simulink model "Solar_power_generation_for_home"  (R2020a)
settings: Solver=VariableStepAuto  StartTime=0.0  StopTime=10.0  RelTol=1e-3
libraries: powerlib x13, powerlib_meascontrol x1, re_lib x1
settings Model: Creator=Reaga  LastModifiedBy=Reaga
settings DebuggingCC: UnconnectedInputMsg=none  UnconnectedOutputMsg=none  UnconnectedLineMsg=none
settings ModelReferenceCC: EnableRefExpFcnMdlSchedulingChecks=off
settings RTWCC: Description=Generic Real-Time Target
settings ConfigComp: CovBoundaryAbsTol=1.0e-5

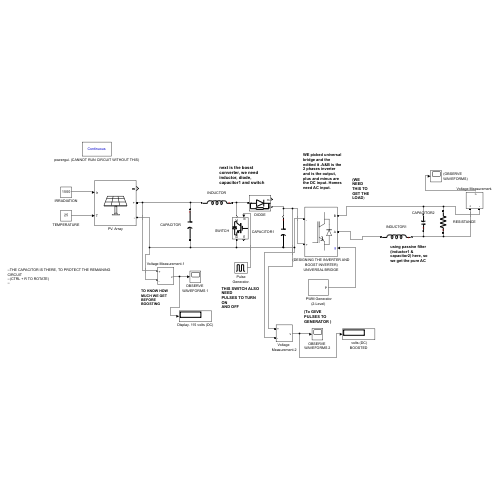
[thumbnail: Simulink's stored preview of the top-level diagram]
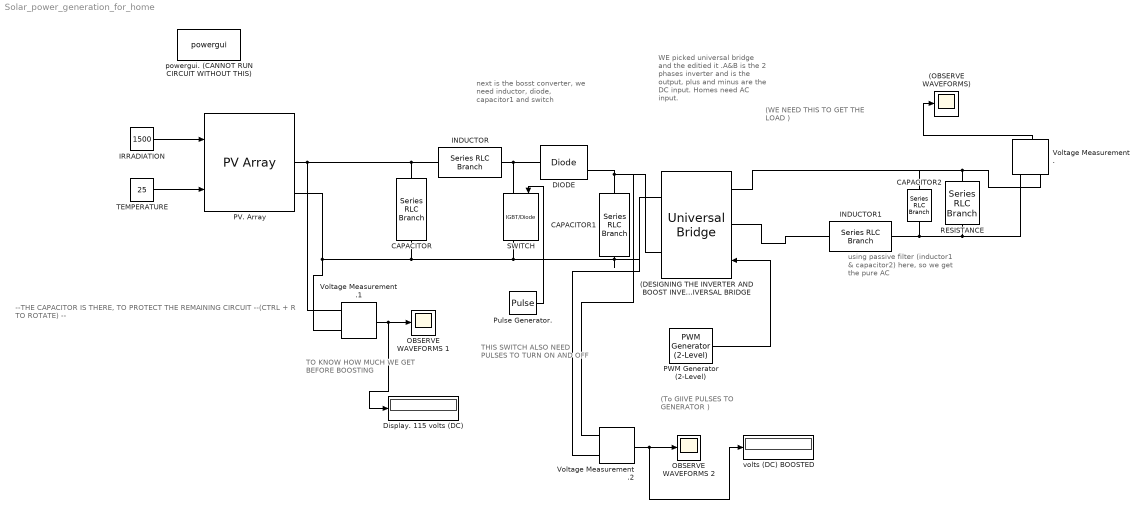
== system Solar_power_generation_for_home ==
  note: using passive filter (inductor1 & capacitor2) here, so we get the pure AC
  note: TO KNOW HOW MUCH WE GET
      | BEFORE BOOSTING
  note: THIS SWITCH ALSO NEED
      | PULSES TO TURN ON
      | AND OFF
  note: (To GIIVE PULSES TO GENERATOR )
  note: (WE NEED THIS TO
      | GET THE LOAD )
  note: WE picked universal bridge and the editied it .A&B is the 2 phases inverter and is the output, plus and minus are the DC input. Homes need AC input.
  note: next is the bosst converter, we need inductor, diode, capacitor1 and switch
  note: --THE CAPACITOR IS THERE, TO PROTECT THE REMAINING CIRCUIT
      | --(CTRL + R TO ROTATE)
      | --
  " SWITCH " : powerlib/Power Electronics/IGBT//Diode  Ron=1e-3  Rs=1e5  Cs=inf  Measurements=on
  " PWM Generator (2-Level)" : powerlib_meascontrol/Pulse & Signal Generators/PWM Generator (2-Level)  ModulatorType=Single-phase full-bridge (4 pulses)  ModulatorMode=Unsynchronized  Fc=27*60  Pc=90  nF=27  MinMax="[ -1  1 ]"  SamplingTechnique=Natural  ModulatingSignals=on  m=0.8  Freq=60  Phase=0  Ts=0  ShowCarrierOutport=off
  " volts (DC) BOOSTED" : Display
  (DESIGNING THE INVERTER AND BOOST INVERTER) UNIVERSAL BRIDGE : powerlib/Power Electronics/Universal Bridge  Arms=2  SnubberResistance=1e5  SnubberCapacitance=inf  Device=IGBT / Diodes  Ron=1e-3  Lon=0  ForwardVoltages="[  0  0  ]"  ForwardVoltage=0  GTOparameters=[ 10e-6 , 20e-6 ]  IGBTparameters=[ 1e-6 , 2e-6 ]  Measurements=None  Measurements_2=None  converterType=Rectifier
  (OBSERVE WAVEFORMS) : Scope
  CAPACITOR : powerlib/Elements/Series RLC Branch  LConnTagsString=__new0  RConnTagsString=__new0  BranchType=C  Resistance=1  Inductance=1e-3  SetiL0=off  InitialCurrent=0  Capacitance=0.006  Setx0=off  InitialVoltage=0  Measurements=None
  CAPACITOR1 : powerlib/Elements/Series RLC Branch  LConnTagsString=__new0  RConnTagsString=__new0  BranchType=C  Resistance=1  Inductance=1e-3  SetiL0=off  InitialCurrent=0  Capacitance=0.006  Setx0=off  InitialVoltage=0  Measurements=None
  CAPACITOR2 : powerlib/Elements/Series RLC Branch  LConnTagsString=__new0  RConnTagsString=__new0  BranchType=C  Resistance=1  Inductance=1e-3  SetiL0=off  InitialCurrent=0  Capacitance=0.006  Setx0=off  InitialVoltage=0  Measurements=None
  DIODE : powerlib/Power Electronics/Diode  Ron=0.001  Lon=0  Vf=0.8  IC=0  UseSnubber=0  Rs=500  Cs=250e-9  Measurements=on
  Display. 115 volts (DC) : Display
  INDUCTOR : powerlib/Elements/Series RLC Branch  LConnTagsString=__new0  RConnTagsString=__new0  BranchType=L  Resistance=1  Inductance=0.02  SetiL0=off  InitialCurrent=0  Capacitance=0.006  Setx0=off  InitialVoltage=0  Measurements=None
  INDUCTOR1 : powerlib/Elements/Series RLC Branch  LConnTagsString=__new0  RConnTagsString=__new0  BranchType=L  Resistance=1  Inductance=0.02  SetiL0=off  InitialCurrent=0  Capacitance=0.006  Setx0=off  InitialVoltage=0  Measurements=None
  IRRADIATION : Constant  Value=1500
  OBSERVE WAVEFORMS 1 : Scope
  OBSERVE WAVEFORMS 2 : Scope
  PV. Array : re_lib/Solar/PV Array  Npar=20  Nser=5  PlotType=array @ 1000 W/m2 & specified temperatures  S_vec="[ 1000  500  100 ]"  Temp_C_vec="[ 45 25  ]"  ModuleName=User-defined  PlotWhenSelected=off  Pm=213.15  Ncell=60  Voc=36.3  Isc=7.84  Vm=29  Im=7.35  beta_Voc_pc=-0.36099  alpha_Isc_pc=0.102  beta_Voc=-0.13104  alpha_Isc=0.0079968  IL=7.8654  I0=2.9273e-10  nI=0.98119  Rsh=313.0553  Rs=0.39381  RobustModel=off  RobustCellTemperature=313.3991  BAL=on  Tc=1e-6  Tfilter=5e-5
  Pulse Generator. : DiscretePulseGenerator  PulseType=Time based  Period=1/1500  PulseWidth=50
  RESISTANCE : powerlib/Elements/Series RLC Branch  LConnTagsString=__new0  RConnTagsString=__new0  BranchType=R  Resistance=1  Inductance=1e-3  SetiL0=off  InitialCurrent=0  Capacitance=0.006  Setx0=off  InitialVoltage=0  Measurements=None
  TEMPERATURE : Constant  Value=25
  Voltage Measurement.2 : powerlib/Measurements/Voltage Measurement  PhasorSimulation=off  OutputType=Complex  PSBequivalent=0
  Voltage Measurement. : powerlib/Measurements/Voltage Measurement  PhasorSimulation=off  OutputType=Complex  PSBequivalent=0
  Voltage Measurement.1 : powerlib/Measurements/Voltage Measurement  PhasorSimulation=off  OutputType=Complex  PSBequivalent=0
  powergui. (CANNOT RUN CIRCUIT WITHOUT THIS) : powerlib/powergui  Priority=1  SimulationMode=Continuous  SampleTime=50e-6  frequency=60  Iterations=50  frequencyindice=0  Pbase=100e6  ErrMax=1e-4  UnitsV=kV  UnitsW=MW  buscounter=0  FunctionMessages=off  echomessages=off  EnableUseOfTLC=off  CurrentSourceSwitches=off  DisableSnubberDevices=off  DisableRonSwitches=off  DisableVfSwitches=off  DisplayEquations=off  AutomaticDiscreteSolvers=off  SolverType=Tustin/Backward Euler (TBE)  Interpol=off  ExternalGateDelay=off  methode=off  Ts=100  x0status=blocks  SPID=on  SwTol=0  HookPort=off  NonlinearTolerance=1e-4  nMaxIteration=100  ContinueOnMaxIteration=off  RestoreLinks=warning  ResistiveCurrentMeasurement=off  Frange=[0:2:500]  Ylog=off  Xlog=on  ShowGrid=off  save=off  variable=ZData  structure=0  ZoomFFT=off  StartTime=0.0  cycles=1  DisplayStyle=1  fundamental=60  FreqAxis=off  MaxFrequency=1000  frequencyindicesteady=1  RmsSteady=1  display=off
  wires:
  TEMPERATURE/1 -> PV. Array/2
  IRRADIATION/1 -> PV. Array/1
  " PWM Generator (2-Level)"/1 -> (DESIGNING THE INVERTER AND BOOST INVERTER) UNIVERSAL BRIDGE/1
  Voltage Measurement./1 -> (OBSERVE WAVEFORMS)/1
  Pulse Generator./1 -> " SWITCH "/1
  Voltage Measurement.1/1 -> Display. 115 volts (DC)/1, OBSERVE WAVEFORMS 1/1
  Voltage Measurement.2/1 -> " volts (DC) BOOSTED"/1, OBSERVE WAVEFORMS 2/1
  connections:
  CAPACITOR/LConn1 -- INDUCTOR/RConn1 -- Voltage Measurement.1/LConn1 -- PV. Array/RConn1
  PV. Array/RConn2 -- Voltage Measurement.1/LConn2 -- (DESIGNING THE INVERTER AND BOOST INVERTER) UNIVERSAL BRIDGE/RConn2 -- Voltage Measurement.2/LConn2 -- CAPACITOR1/RConn1 -- " SWITCH "/RConn1 -- CAPACITOR/RConn1
  DIODE/LConn1 -- " SWITCH "/LConn1 -- INDUCTOR/LConn1
  RESISTANCE/LConn1 -- CAPACITOR2/LConn1 -- INDUCTOR1/LConn1 -- Voltage Measurement./LConn1
  RESISTANCE/RConn1 -- CAPACITOR2/RConn1 -- (DESIGNING THE INVERTER AND BOOST INVERTER) UNIVERSAL BRIDGE/LConn2 -- Voltage Measurement./LConn2
  DIODE/RConn1 -- Voltage Measurement.2/LConn1 -- (DESIGNING THE INVERTER AND BOOST INVERTER) UNIVERSAL BRIDGE/RConn1 -- CAPACITOR1/LConn1
  INDUCTOR1/RConn1 -- (DESIGNING THE INVERTER AND BOOST INVERTER) UNIVERSAL BRIDGE/LConn1
